simulink model "turtletrajectory"  (R2018b)
settings: Solver=FixedStepAuto  StartTime=0.0  StopTime=inf  FixedStep=0.01  RelTol=1e-3
undefined symbols (not defined in the file or in its folder): Angular, Linear
libraries: simulink x4, robotlib x3
settings Model: Creator=DwigHT  LastModifiedBy=DwigHT
settings OptimizationCC: EnhancedBackFolding=on  PassReuseOutputArgsAs=Individual arguments  MaxStackSize=64  OptimizeBlockOrder=speed  DifferentSizesBufferReuse=on  OptimizationCustomize=off
settings DebuggingCC: ParameterTunabilityLossMsg=error
settings HardwareCC: ProdBitPerPointer=32  ProdBitPerSizeT=32  ProdBitPerPtrDiffT=32  ProdLargestAtomicFloat=None  ProdIntDivRoundTo=Undefined  ProdEndianess=Unspecified  ProdWordSize=32  ProdHWDeviceType=Generic->Unspecified (assume 32-bit Generic)
settings SFSimCC: MATLABDynamicMemAlloc=off
settings RTWCC: SystemTargetFile=ert.tlc  HardwareBoard=Robot Operating System (ROS)  TLCOptions="-aInlineSetEventsForThisBaseRateFcn=TLC_FALSE -aSuppressMultiTaskScheduler=TLC_FALSE  -aRateBasedStepFcn=0"  TemplateMakefile=ert_default_tmf  GenerateReport=on  Toolchain=Catkin  IncludeHyperlinkInReport=on  LaunchReport=on  TargetLang=C++  GenerateTraceInfo=on  GenerateTraceReport=on  GenerateTraceReportSl=on  GenerateTraceReportSf=on  GenerateTraceReportEml=on
settings CodeAppCC: ForceParamTrailComments=on  IgnoreCustomStorageClasses=off  OperatorAnnotations=on  SimulinkDataObjDesc=on  SFDataObjDesc=on  InsertBlockDesc=on

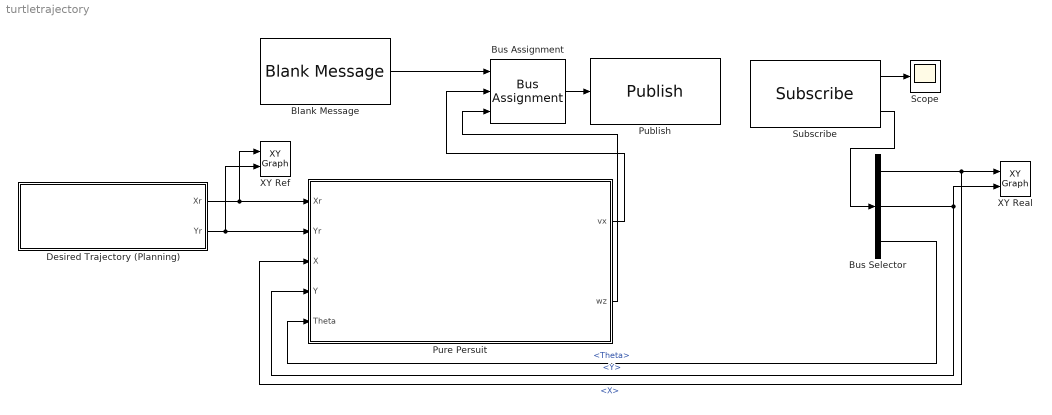
== system turtletrajectory ==
  Blank Message : robotlib/Blank Message  messageClass=Message  entityType=geometry_msgs/Twist  messageType=geometry_msgs/Twist  SampleTime=inf
      settings: SourceProductBaseCode=RO
  Bus Assignment : BusAssignment  AssignedSignals=Linear.X,Angular.Z
  Bus Selector : BusSelector  OutputSignals=X,Y,Theta
  Desired Trajectory (Planning) : Subsystem
  Publish : robotlib/Publish  topicSource=Select from ROS network  topic=/turtle1/cmd_vel  messageType=geometry_msgs/Twist  messageQueueLength=1
      settings: SourceProductBaseCode=RO
  Pure Persuit : Subsystem
  Scope : Scope
  Subscribe : robotlib/Subscribe  topicSource=Select from ROS network  topic=/turtle1/pose  messageType=turtlesim/Pose  sampleTime=-1  messageQueueLength=1
      settings: SourceProductBaseCode=RO
  XY Real : simulink/Sinks/XY Graph  xmin=0  xmax=11  ymin=0  ymax=11  st=-1
  XY Ref : simulink/Sinks/XY Graph  xmin=0  xmax=11  ymin=0  ymax=11  st=-1
  wires:
  Desired Trajectory (Planning)/1(Xr) -> XY Ref/1, Pure Persuit/1(Xr)
  Desired Trajectory (Planning)/2(Yr) -> XY Ref/2, Pure Persuit/2(Yr)
  Bus Selector/2 -> Pure Persuit/4(Y), XY Real/2  "<Y>"
  Bus Selector/1 -> Pure Persuit/3(X), XY Real/1  "<X>"
  Bus Selector/3 -> Pure Persuit/5(Theta)  "<Theta>"
  Pure Persuit/1(vx) -> Bus Assignment/2
  Pure Persuit/2(wz) -> Bus Assignment/3
  Subscribe/2 -> Bus Selector/1
  Subscribe/1 -> Scope/1
  Blank Message/1 -> Bus Assignment/1
  Bus Assignment/1 -> Publish/1

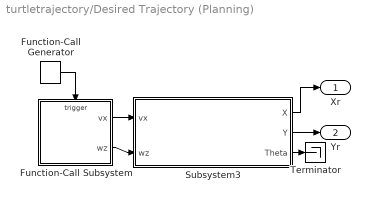
== system turtletrajectory/Desired Trajectory (Planning) ==
  Function-Call Generator : simulink/Ports & Subsystems/Function-Call Generator  sample_time=1  numberOfIterations=1
  Function-Call Subsystem : Subsystem  TreatAsAtomicUnit=on
  Subsystem3 : Subsystem
  Terminator : Terminator
  Xr : Outport
  Yr : Outport  Port=2
  wires:
  Subsystem3/2(Y) -> Yr/1
  Subsystem3/3(Theta) -> Terminator/1
  Function-Call Subsystem/2(wz) -> Subsystem3/2(wz)
  Function-Call Subsystem/1(vx) -> Subsystem3/1(vx)
  Subsystem3/1(X) -> Xr/1
  Function-Call Generator/1 -> Function-Call Subsystem/Trigger

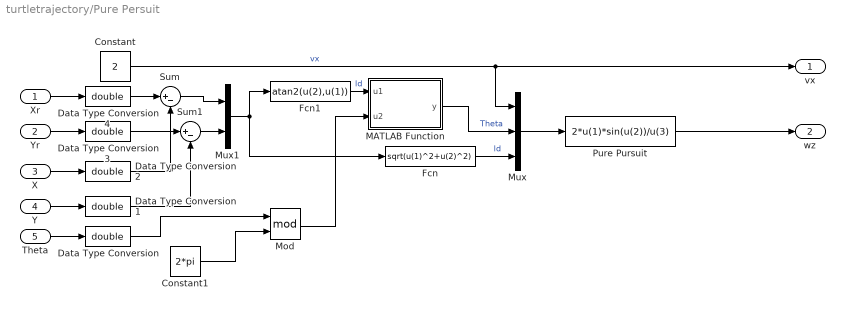
== system turtletrajectory/Pure Persuit ==
  Xr : Inport
  Yr : Inport  Port=2
  X : Inport  Port=3
  Y : Inport  Port=4
  Theta : Inport  Port=5
  Constant : Constant  Value=2
  Constant1 : Constant  Value=2*pi
  Data Type Conversion{,1..4} (5 alike) : DataTypeConversion  OutDataTypeStr=double
  Fcn : Fcn  Expr=sqrt(u(1)^2+u(2)^2)
  Fcn1 : Fcn  Expr=atan2(u(2),u(1))
  MATLAB Function : MATLAB Function  TreatAsAtomicUnit=on
  Mod : Math  Operator=mod  SaturateOnIntegerOverflow=on
  Mux : Mux  Inputs=3
  Mux1 : Mux  Inputs=2
  Pure Pursuit : Fcn  Expr=2*u(1)*sin(u(2))/u(3)
  Sum : Sum  Inputs=|+-
  Sum1 : Sum  Inputs=|+-
  vx : Outport
  wz : Outport  Port=2
  wires:
  Mux/1 -> Pure Pursuit/1
  Sum1/1 -> Mux1/2
  Fcn1/1 -> MATLAB Function/1(u1)  "ld"
  Constant/1 -> vx/1, Mux/1  "vx"
  Mod/1 -> MATLAB Function/2(u2)
  Sum/1 -> Mux1/1
  MATLAB Function/1(y) -> Mux/2  "Theta"
  Mux1/1 -> Fcn1/1, Fcn/1
  Constant1/1 -> Mod/2
  Fcn/1 -> Mux/3  "ld"
  Yr/1 -> Data Type Conversion3/1
  Xr/1 -> Data Type Conversion4/1
  X/1 -> Data Type Conversion2/1
  Y/1 -> Data Type Conversion1/1
  Theta/1 -> Data Type Conversion/1
  Pure Pursuit/1 -> wz/1
  Data Type Conversion/1 -> Mod/1
  Data Type Conversion1/1 -> Sum1/2
  Data Type Conversion2/1 -> Sum/2
  Data Type Conversion3/1 -> Sum1/1
  Data Type Conversion4/1 -> Sum/1

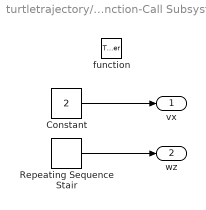
== system turtletrajectory/Desired Trajectory (Planning)/Function-Call Subsystem ==
  function : TriggerPort  TriggerType=function-call  VariantControl=Variant
  Constant : Constant  Value=2
  Repeating Sequence Stair : simulink/Sources/Repeating Sequence Stair  OutValues=[1 2 3 2].'  tsamp=-1  OutMin=[]  OutMax=[]  OutDataTypeStr=double  OutputDataTypeScalingMode=double  OutDataType=fixdt(0,8)  ConRadixGroup=Best Precision: Vector-wise  OutScaling=2^-12
  vx : Outport
  wz : Outport  Port=2
  wires:
  Constant/1 -> vx/1
  Repeating Sequence Stair/1 -> wz/1

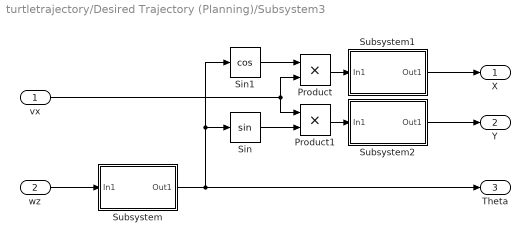
== system turtletrajectory/Desired Trajectory (Planning)/Subsystem3 ==
  vx : Inport
  wz : Inport  Port=2
  Product : Product
  Product1 : Product
  Sin : Trigonometry
  Sin1 : Trigonometry  Operator=cos
  Subsystem : Subsystem
  Subsystem1 : Subsystem
  Subsystem2 : Subsystem
  X : Outport
  Y : Outport  Port=2
  Theta : Outport  Port=3
  wires:
  Product1/1 -> Subsystem2/1(In1)
  Subsystem2/1(Out1) -> Y/1
  Sin1/1 -> Product/1
  Subsystem1/1(Out1) -> X/1
  vx/1 -> Product/2, Product1/1
  Product/1 -> Subsystem1/1(In1)
  Subsystem/1(Out1) -> Theta/1, Sin/1, Sin1/1
  Sin/1 -> Product1/2
  wz/1 -> Subsystem/1(In1)

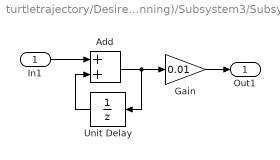
== system turtletrajectory/Desired Trajectory (Planning)/Subsystem3/Subsystem ==
  In1 : Inport
  Add : Sum
  Gain : Gain  Gain=0.01
  Unit Delay : UnitDelay  SampleTime=0.01
  Out1 : Outport
  wires:
  Unit Delay/1 -> Add/2
  Add/1 -> Gain/1, Unit Delay/1
  Gain/1 -> Out1/1
  In1/1 -> Add/1

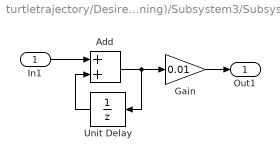
== system turtletrajectory/Desired Trajectory (Planning)/Subsystem3/Subsystem1 ==
  In1 : Inport
  Add : Sum
  Gain : Gain  Gain=0.01
  Unit Delay : UnitDelay  InitialCondition=555  SampleTime=0.01
  Out1 : Outport
  wires:
  In1/1 -> Add/1
  Gain/1 -> Out1/1
  Add/1 -> Unit Delay/1, Gain/1
  Unit Delay/1 -> Add/2

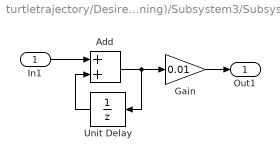
== system turtletrajectory/Desired Trajectory (Planning)/Subsystem3/Subsystem2 ==
  In1 : Inport
  Add : Sum
  Gain : Gain  Gain=0.01
  Unit Delay : UnitDelay  InitialCondition=555  SampleTime=0.01
  Out1 : Outport
  wires:
  Unit Delay/1 -> Add/2
  Add/1 -> Gain/1, Unit Delay/1
  Gain/1 -> Out1/1
  In1/1 -> Add/1

== matlab function turtletrajectory/Pure Persuit/MATLAB Function ==
  data: u1 input; y output; u2 input
function y = fcn(u1,u2)
if u1<0
    u1=u1+2*pi;
end
y = u1-u2;
